simulink model "cell_balance"  (R2022b)
settings: Solver=FixedStepDiscrete  StartTime=0.0  StopTime=10.0  FixedStep=1e-3  MaxStep=1e-3  RelTol=1e-3
undefined symbols (not defined in the file or in its folder): BMS_mode
(part 2 of 2)

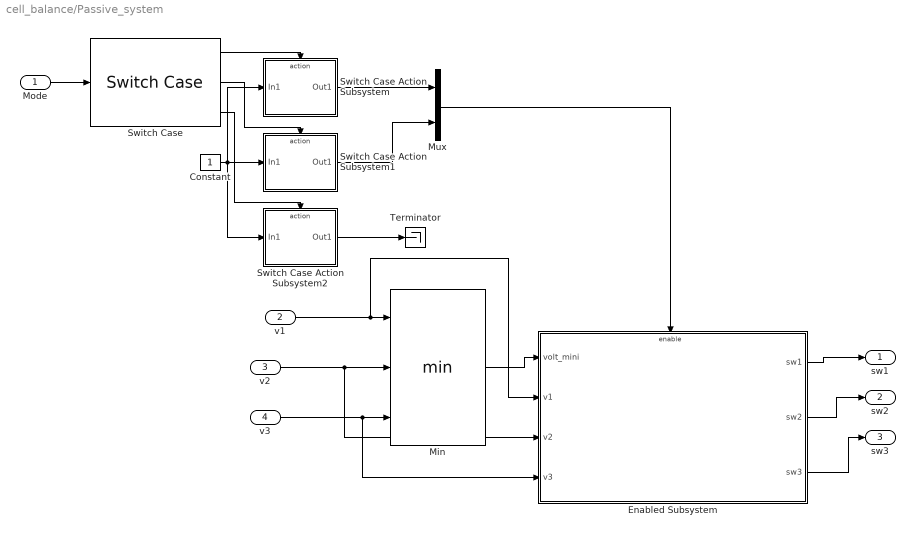
== system cell_balance/Passive_system ==
  Mode : Inport
  v1 : Inport  Port=2
  v2 : Inport  Port=3
  v3 : Inport  Port=4
  Constant : Constant
  Enabled Subsystem : Subsystem  TreatAsAtomicUnit=on
  Min : MinMax  Inputs=3
  Mux : Mux  Inputs=2
  Switch Case : SwitchCase  CaseConditions=[BMS_mode.off,BMS_mode.charging,BMS_mode.discharging]  ShowDefaultCase=off
  Switch Case Action Subsystem : Subsystem  TreatAsAtomicUnit=on
  Switch Case Action Subsystem1 : Subsystem  TreatAsAtomicUnit=on
  Switch Case Action Subsystem2 : Subsystem  TreatAsAtomicUnit=on
  Terminator : Terminator
  sw1 : Outport
  sw2 : Outport  Port=2
  sw3 : Outport  Port=3
  wires:
  v3/1 -> Enabled Subsystem/4(v3), Min/3
  v1/1 -> Enabled Subsystem/2(v1), Min/1
  Mode/1 -> Switch Case/1
  Switch Case Action Subsystem1/1(Out1) -> Mux/2
  Mux/1 -> Enabled Subsystem/Enable
  Switch Case/1 -> Switch Case Action Subsystem/Action
  Switch Case Action Subsystem/1(Out1) -> Mux/1
  Switch Case/2 -> Switch Case Action Subsystem1/Action
  Switch Case/3 -> Switch Case Action Subsystem2/Action
  Switch Case Action Subsystem2/1(Out1) -> Terminator/1
  Constant/1 -> Switch Case Action Subsystem2/1(In1), Switch Case Action Subsystem1/1(In1), Switch Case Action Subsystem/1(In1)
  v2/1 -> Enabled Subsystem/3(v2), Min/2
  Min/1 -> Enabled Subsystem/1(volt_mini)
  Enabled Subsystem/2(sw2) -> sw2/1
  Enabled Subsystem/1(sw1) -> sw1/1
  Enabled Subsystem/3(sw3) -> sw3/1

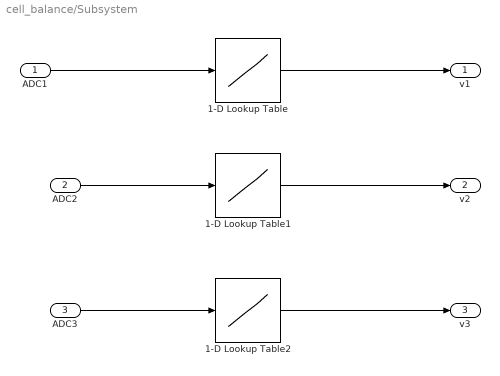
== system cell_balance/Subsystem ==
  ADC1 : Inport
  ADC2 : Inport  Port=2
  ADC3 : Inport  Port=3
  1-D Lookup Table : Lookup_n-D  NumberOfTableDimensions=1  LookupTableObject=''  BreakpointsForDimension1=int16([347,406,570,722,901,1101,1344,1434,1671,1785,1937,2139])  BreakpointsForDimension1FirstPoint=10  BreakpointsForDimension2FirstPoint=10  BreakpointsForDimension1Spacing=12  BreakpointsForDimension2Spacing=12  Table=single([0.11,0.28,0.72,1.13,1.61,2.16,2.84,3.11,3.77,4.1,4.53,5.12])  InterpMethod=Cubic spline  ExtrapMethod=Cubic spline  DiagnosticForOutOfRangeInput=Error  InternalRulePriority=Speed  RndMeth=Simplest
  1-D Lookup Table1 : Lookup_n-D  NumberOfTableDimensions=1  LookupTableObject=''  BreakpointsForDimension1=int16([364,468,633,845,1028,1094,1264,1457,1591,1826,1943,2126,2215])  BreakpointsForDimension1FirstPoint=10  BreakpointsForDimension2FirstPoint=10  BreakpointsForDimension1Spacing=12  BreakpointsForDimension2Spacing=12  Table=single([0.08,0.36,0.78,1.33,1.81,1.98,2.44,2.97,3.34,3.97,4.29,4.79,5.02])  InterpMethod=Cubic spline  ExtrapMethod=Cubic spline  DiagnosticForOutOfRangeInput=Error  InternalRulePriority=Speed  RndMeth=Simplest
  1-D Lookup Table2 : Lookup_n-D  NumberOfTableDimensions=1  LookupTableObject=''  BreakpointsForDimension1=int16([286,662,795,948,1112,1228,1493,1705,1965,2172])  BreakpointsForDimension1FirstPoint=10  BreakpointsForDimension2FirstPoint=10  BreakpointsForDimension1Spacing=12  BreakpointsForDimension2Spacing=12  Table=single([0.06,1.06,1.39,1.80,2.20,2.51,3.08,3.57,4.21,4.75])  InterpMethod=Cubic spline  ExtrapMethod=Cubic spline  DiagnosticForOutOfRangeInput=Error  InternalRulePriority=Speed  RndMeth=Simplest
  v1 : Outport
  v2 : Outport  Port=2
  v3 : Outport  Port=3
  wires:
  1-D Lookup Table/1 -> v1/1
  ADC1/1 -> 1-D Lookup Table/1
  ADC2/1 -> 1-D Lookup Table1/1
  1-D Lookup Table1/1 -> v2/1
  1-D Lookup Table2/1 -> v3/1
  ADC3/1 -> 1-D Lookup Table2/1

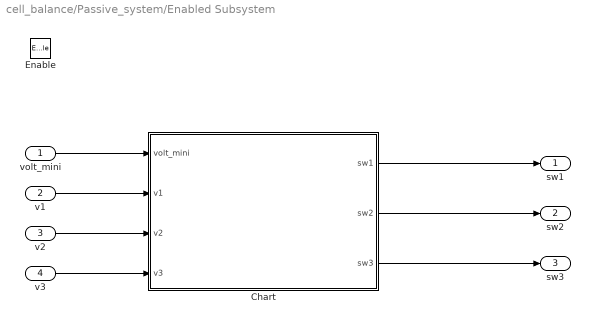
== system cell_balance/Passive_system/Enabled Subsystem ==
  volt_mini : Inport
  v1 : Inport  Port=2
  v2 : Inport  Port=3
  v3 : Inport  Port=4
  Enable : EnablePort
  Chart : Stateflow chart  TreatAsAtomicUnit=on
      settings: PortSchema="{\"entries\":[{\"content\":{\"sides\":[{\"content\":{\"connectorIds\":[\"In1\",\"In2\",\"In3\",\"In4\"]},\"type\":\"ConnectorPlacement.EquallySpacedRectSide\",\"uuid\":\"f29a8cda-8803-475f-abd3-4e4339aba25e\"},{\"content\":{\"connectorIds\":[\"Out2\",\"Out3\",\"Out1\"],\"side\":\"RIGHT\"},\"type\":\"ConnectorPlacement.EquallySpacedRectSide\",\"uuid\":\"0598b39c-caa4-4adf-8d5c-28c07f0296f4\"},{\"content\":{\"connectorIds\":[],\"side\":\"TOP\"},\"type\":\"ConnectorPlacement.EquallySpacedRectSide\",\"uuid\":\"9f38f119-9f27-4a8e-b2cb-7c7e66af6571\"},{\"content\":{\"connectorIds\":[],\"side\":\"BOTTOM\"},\"type\":\"ConnectorPlacement.EquallySpacedRectSide\",\"uuid\":\"32b45aed-3993-4991-a8ea-fcd5247e15e7\"}]},\"type\":\"ConnectorPlacement.EquallySpacedConnector\",\"uuid\":\"c85bfddf-40ea-4a5b-9c2d-94a149e11b52\"}],\"packageUris\":[\"http://schema.mathworks.com/mf0/Connector/R2020b\"],\"version\":\"1.0\"}"
  sw1 : Outport
  sw2 : Outport  Port=2
  sw3 : Outport  Port=3
  wires:
  volt_mini/1 -> Chart/1(volt_mini)
  Chart/2(sw1) -> sw1/1
  Chart/3(sw2) -> sw2/1
  Chart/1(sw3) -> sw3/1
  v1/1 -> Chart/2(v1)
  v2/1 -> Chart/3(v2)
  v3/1 -> Chart/4(v3)

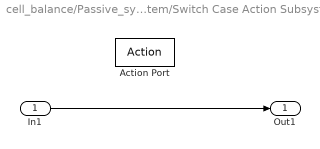
== system cell_balance/Passive_system/Switch Case Action Subsystem ==
  In1 : Inport
  Action Port : ActionPort  ActionPortLabel=case [ off ]:
  Out1 : Outport
  wires:
  In1/1 -> Out1/1

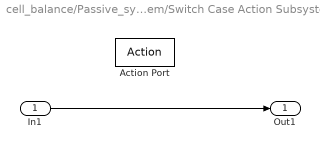
== system cell_balance/Passive_system/Switch Case Action Subsystem1 ==
  In1 : Inport
  Action Port : ActionPort  ActionPortLabel=case [ charging ]:
  Out1 : Outport
  wires:
  In1/1 -> Out1/1

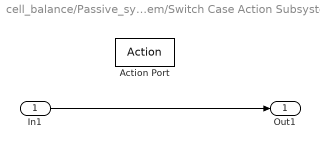
== system cell_balance/Passive_system/Switch Case Action Subsystem2 ==
  In1 : Inport
  Action Port : ActionPort  ActionPortLabel=case [ discharging ]:
  Out1 : Outport
  wires:
  In1/1 -> Out1/1

== stateflow chart cell_balance/Passive_system/Enabled Subsystem/Chart ==
  (default) -> (junction 20)
  (junction 20) -> (junction 21) [order 1] : [(volt_mini==v1) ]
  (junction 20) -> (junction 181) [order 2]
  (junction 21) -> (junction 29) : {sw2=1; sw3=1; }
  (junction 181) -> (junction 182) [order 1] : [ (volt_mini==v1)  && ( v2 == (v1 +0.1) ) ]
  (junction 181) -> (junction 22) [order 2]
  (junction 182) -> (junction 183) : {sw2=0;}
  (junction 22) -> (junction 23) [order 1] : [(volt_mini==v1)  && ( v3  == (v1 +0.1) )]
  (junction 22) -> (junction 26) [order 2]
  (junction 23) -> (junction 28) : { sw3=0;}
  (junction 28) -> (junction 26)
  (junction 183) -> (junction 28)
  (junction 29) -> (junction 183)
  (junction 26) -> (junction 48)
  (junction 48) -> (junction 44) [order 1] : [(volt_mini==v2)]
  (junction 48) -> (junction 190) [order 2]
  (junction 44) -> (junction 64) : {sw1=1; sw3=1; }
  (junction 190) -> (junction 191) [order 2] : [(volt_mini==v2)  &&  (v1 == (v2 +0.1) )]
  (junction 190) -> (junction 42) [order 1]
  (junction 191) -> (junction 192) : {sw1=0;}
  (junction 42) -> (junction 43) [order 1] : [(volt_mini==v2)  && ( v3 == (v2 +0.1) )]
  (junction 42) -> (junction 45) [order 2]
  (junction 43) -> (junction 49) : { sw3=0;}
  (junction 192) -> (junction 49)
  (junction 64) -> (junction 192)
  (junction 49) -> (junction 45)
  (junction 45) -> (junction 120)
  (junction 120) -> (junction 111) [order 1] : [(volt_mini==v3)]
  (junction 120) -> (junction 199) [order 2]
  (junction 111) -> (junction 96) : {sw1=1; sw2=1; }
  (junction 199) -> (junction 200) [order 1] : [(volt_mini==v3)  && ( v1 == (v3 +0.1) )]
  (junction 199) -> (junction 117) [order 2]
  (junction 200) -> (junction 201) : {sw1=0;}
  (junction 117) -> (junction 116) [order 1] : [(volt_mini==v3)  && ( v2 == (v3 +0.1) )]
  (junction 117) -> (junction 109) [order 2]
  (junction 116) -> (junction 114) : {sw2=0;}
  (junction 201) -> (junction 114)
  (junction 96) -> (junction 201)
  (junction 114) -> (junction 109)
  (junction 109) -> (junction 208)
  data: sw3 output; volt_mini input; sw1 output; sw2 output; v1 input; v2 input; v3 input
